simulink model "disco"  (R2015a)
settings: Solver=ode45  StartTime=0.0  StopTime=10.0  RelTol=1e-3
undefined symbols (not defined in the file or in its folder): sgn
settings Model: Creator=abran  LastModifiedBy=abran

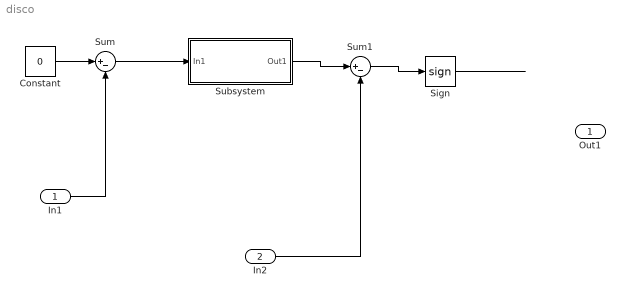
== system disco ==
  In1 : Inport
  In2 : Inport  Port=2
  Constant : Constant  Value=0
  Sign : Signum
  Subsystem : Subsystem
  Sum : Sum  Inputs=|+-
  Sum1 : Sum  Inputs=|+-
  Out1 : Outport
  wires:
  Constant/1 -> Sum/1
  Sum/1 -> Subsystem/1(In1)
  Subsystem/1(Out1) -> Sum1/1
  Sum1/1 -> Sign/1
  Sign/1 -> ?
  In1/1 -> Sum/2
  In2/1 -> Sum1/2

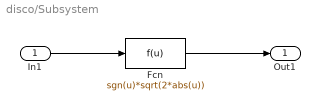
== system disco/Subsystem ==
  In1 : Inport
  Fcn : Fcn  Expr=sgn(u)*sqrt(2*abs(u))
  Out1 : Outport
  wires:
  In1/1 -> Fcn/1
  Fcn/1 -> Out1/1
